simulink model "ssc_auto_ev_20b"  (R2020b)
settings: Solver=VariableStepAuto  StartTime=0.0  StopTime=200  RelTol=1e-3  AbsTol=1e-3
PreLoadFcn:
  | % Simulation parameters
  | dt = 0.01;
  | 
  | % Battery cell parameters
  | ssc_lithium_cell_1RC_ini
  | Nseries = 100;
  | Nparallel = 10;
  | 
  | % Motor parameters
  | max_torque = 220;
  | max_power = 80e3;
  | 
  | % Vehicle parameters
  | vehicle_mass = 4000;
  | wheel_radius = 0.35;
  | area = 5;
  | drag_coefficient = 0.25;
  | air_density = 1.225;
  | gravity = 9.81;
  | rolling_res_ratio = 0.015;
  | 
  | % Differential drive parameters
  | gear_ratio = 12;
  | 
  | % Simplified braking system parameters
  | force_max_pedal = 500;
  | braking_torque_to_pedal_force_ratio = -16;
  | 
  | % Vehicle controller parameters
  | hill_hold_max_speed = 0.5;
  | 
  | % Water properties for cooling circuit
  | load WaterProperties
  | 
  | % Input signals for Signal Editor block
  | load ssc_auto_ev_Inputs
values from neighbouring files (symbols this model uses):
  C1_LUT = [1913.6 4625.7 23306 10736 18036 12251 9022.9 12447 18872 40764 18721 33630 ... (21 elements, 7x3)]    [ssc_auto_ev_param.mat]
  Capacity_LUT = [28.0081 27.625 27.6392]    [ssc_auto_ev_param.mat]
  cell_Cp_heat = 810.5328    [ssc_auto_ev_param.mat]
  cell_mass = 1    [ssc_auto_ev_param.mat]
  Em_LUT = [3.4966 3.5519 3.6183 3.7066 3.9131 4.0748 4.1923 3.5057 3.566 3.6337 3.7127 3.9259 ... (21 elements, 7x3)]    [ssc_auto_ev_param.mat]
  Qe_init = 15.6845    [ssc_auto_ev_param.mat]
  R0_LUT = [0.0117 0.011 0.0114 0.0107 0.0107 0.0113 0.0116 0.0085 0.0085 0.0087 0.0082 0.0083 ... (21 elements, 7x3)]    [ssc_auto_ev_param.mat]
  R1_LUT = [0.0109 0.0069 0.0047 0.0034 0.0033 0.0033 0.0028 0.0029 0.0024 0.0026 0.0016 0.0023 ... (21 elements, 7x3)]    [ssc_auto_ev_param.mat]
  SOC_LUT = [0 0.1 0.25 0.5 0.75 0.9 1]    [ssc_auto_ev_param.mat]
  T_init = 293.15    [ssc_auto_ev_param.mat]
  Temperature_LUT = [278.15 293.15 313.15]    [ssc_auto_ev_param.mat]
undefined symbols (not defined in the file or in its folder): DiscIntNeverNeededParam, K, Lambda, tau, x0
libraries: fl_lib x656, nesl_utility x86, simulink x21, LiBatteryElements_lib x16, SignalEditorBlockLib x4, simulink_extras x4
(part 2 of 13)

== system ssc_auto_ev_20b/Step 2: Multirate Model ==
  note: The rotor iron thermal mass was pulled out of the
      | motor thermal model subsystem in Step 1 so that
      | it could be used to separate the thermal network
      | from the rest of the model in Step 2. Here, in Step 2,
      | it is replaced by a thermal mass network coupler
      | block from the Simscape Network Coupliers Library.
      | The same approach is used for the other motor and
      | the battery.
  note: There is no suitable existing model dynamic with
      | which to break the electrical connection to the battery.
      | Hence a network coupler block with internal voltage
      | and current sources is used which introduces its own
      | time constant. The electrical "+" connection of the
      | Motor Drive block has a series-connected current
      | source, and hence the voltage source in the coupler
      | block is connected to this port to avoid an invalid topology.
  note: The thermal circuit is set to run five times slower
      | than the control and vehicle dynamics subsystems.
      | It is often the case that the thermal time constants
      | are slower than the other domain time constants,
      | and so a longer sample time can be used.
  note: The battery subsystem is set to run two
      | times slower than the control and vehicle
      | dynamics subsystems. Battery time constants
      | are also typically slower than drive torque time
      | constants and mechanical time constants, and
      | so can be run with a larger sample time.
  note: Experimenting with the flexible
      | shaft coupler by using its Analysis
      | tab indicates that breaking the
      | network at this rotating shaft
      | is not a good idea. It would
      | require the sampling to be
      | increased to about 1000Hz to
      | track the design model.
  Battery : Subsystem  mask(Lithium cell (one RC-branch equivalent circuit)){Nseries=Nseries, Nparallel=Nparallel, Qe_init=Qe_init, T_init=T_init, Capacity_LUT=Capacity_LUT, Em_LUT=Em_LUT, R0_LUT=R0_LUT, R1_LUT=R1_LUT, C1_LUT=C1_LUT, cell_mass=cell_mass, cell_Cp_heat=cell_Cp_heat, SOC_LUT=SOC_LUT, Temperature_LUT=Temperature_LUT}
      mask prompts: Nseries "Number of series-connected parallel sets"; Nparallel "Number of parallel-connected cells per parallel set"; Qe_init "Initial cell charge deficit (A*hr)"; T_init "Initial cell temperature (K)"; Capacity_LUT "Capacity (A*hr, 1xN table)"; Em_LUT "Em open-circuit voltage, Em (volts, MxN table)"; R0_LUT "R0 terminal resistance (ohms, MxN table)"; R1_LUT "R1 cell resistance (ohms, MxN table)"; C1_LUT "C1 capacitance (farads, MxN table)"; cell_mass "Cell mass (kg)"; cell_Cp_heat "Cell specific heat (J/kg/K)"; SOC_LUT "SOC table breakpoints (Mx1 array)"; Temperature_LUT "Temperature table breakpoints (K, 1xN array)"
      mask DialogControl ParameterTabVar0 Prompt: Main
      mask DialogControl ParameterTabVar01 Prompt: Electrical (per cell)
      mask DialogControl ParameterTabVar012 Prompt: Thermal (per cell)
      mask DialogControl ParameterTabVar0123 Prompt: Table Breakpoints
      mask Display:
      | % Battery icon
      | plot([1.8 1.3],[0 0])
      | plot([-0.6 -1.6 -1.6 -2.2],[0 0 -0.9 -0.9])
      | patch([1 1 -1 -1]*0.15+0.7,[-1 1 1 -1]*0.4,[0;0;0]);
      | patch([1 1 -1 -1]*0.15-0.6,[-1 1 1 -1]*0.4,[0;0;0]);
      | patch([1 1 -1 -1]*0.15+1.3,[-1 1 1 -1]*0.8,[0;0;0]);
      | patch([1 1 -1 -1]*0.15-0.0,[-1 1 1 -1]*0.8,[0;0;0]);
      | % Thermal port
      | plot([-1.6,-1.3],[1.2,1.2])
      | plot([-1.6,-1.3],[0.5,0.5])
      | plot([-1.6,-2.5],[0.8,0.8])
      | plot(0.2*sin(0:2*pi/50:2*pi)-1.6,0.35*cos(0:2*pi/50:2*pi)+0.85)
      | plot(0.2*sin(0:2*pi/50:pi)-1.3,0.35*cos(0:2*pi/50:pi)+0.85)
      | 
      | % Plot points to set plot range
      | color('white');plot(2.5,1.5);plot(-2.5,-1.5)
  Battery Thermal Mass : Subsystem  mask(Network Coupler (Thermal Mass)){}
      mask init:
      | % Icon
      | %key = 'Simscape.NetworkCouplers.ThermalMass';
      | %foundation.internal.couplers.updateIcon(gcb,'thermalMass.svg',key)
      settings: OpenFcn=open_system(gcbh,'force')
      mask Help: web([docroot '/physmod/simscape/ref/networkcouplerthermalmass.html'])
      mask Display:
      | color('red');
      | port_label('LConn', 1,'1')
      | port_label('RConn', 1,'2')
  Cooling System : Subsystem  Tag=PublishSubsystem
      settings: PortSchema="{\"entries\":[{\"content\":{\"sides\":[{\"content\":{\"connectorIds\":[]},\"type\":\"ConnectorPlacement.EquallySpacedRectSide\",\"uuid\":\"d96bbf63-bcbb-4f3a-92bd-eaf78ab4538b\"},{\"content\":{\"connectorIds\":[],\"side\":\"RIGHT\"},\"type\":\"ConnectorPlacement.EquallySpacedRectSide\",\"uuid\":\"b082d3d3-6635-4bf9-9df2-69e4bab78a2b\"},{\"content\":{\"connectorIds\":[\"LConn1\"],\"side\":\"TOP\"},\"type\":\"ConnectorPlacement.EquallySpacedRectSide\",\"uuid\":\"f7177de9-9ba4-478b-b096-87cbc5cd4871\"},{\"content\":{\"connectorIds\":[\"RConn1\"],\"side\":\"BOTTOM\"},\"type\":\"ConnectorPlacement.EquallySpacedRectSide\",\"uuid\":\"4233a269-bfd6-4033-b1ed-0dae7bb50bca\"}]},\"type\":\"ConnectorPlacement.EquallySpacedConnector\",\"uuid\":\"6f10551f-62c9-4564-9ac9-7ef3b87c77d6\"}],\"packageUris\":[\"http://schema.mathworks.com/mf0/Connector/R2020b\"],\"version\":\"1.0\"}"
  Driver and Environment : Subsystem
  ERef1 : fl_lib/Electrical/Electrical Elements/Electrical Reference
      settings: SourceProductBaseCode=PW,SS,VE
  ERef2 : fl_lib/Electrical/Electrical Elements/Electrical Reference
      settings: SourceProductBaseCode=PW,SS,VE
  Environment : Subsystem
  Motor 1 Thermal Model : Subsystem
  Motor 2 Thermal Model : Subsystem
  Motor Drive : Subsystem  Tag=PublishSubsystem  VariantControl=Variant1
  Network Coupler (Flexible Shaft) : Subsystem  Commented=on  mask(Network Coupler (Flexible Shaft)){}
      mask init:
      | % Icon
      | key = 'Simscape.NetworkCouplers.FlexibleShaft';
      | foundation.internal.couplers.updateIcon(gcb,'flexibleShaft.svg',key)
      settings: OpenFcn=open_system(gcbh,'force')
      mask Help: web([docroot '/physmod/simscape/ref/networkcouplerflexibleshaft.html'])
      mask Display:
      | color('red');
      | port_label('LConn', 1,'1')
      | port_label('RConn', 1,'2')
  Network Coupler (Voltage-Current) : Subsystem  mask(Network Coupler (Voltage-Current)){}
      mask init:
      | % Icon
      | %key = 'Simscape.NetworkCouplers.ElectricalVoltageCurrent';
      | %foundation.internal.couplers.updateIcon(gcb,'voltageCurrentSource.svg',key)
      settings: OpenFcn=open_system(gcbh,'force')
      mask Help: web([docroot '/physmod/simscape/ref/networkcouplervoltagecurrent.html'])
      mask Display:
      | color('red');
      | port_label('LConn', 1,'1')
      | port_label('RConn', 1,'2')
  Rotor Iron Thermal Mass/1 : Subsystem  mask(Network Coupler (Thermal Mass)){}
      mask init:
      | % Icon
      | %key = 'Simscape.NetworkCouplers.ThermalMass';
      | %foundation.internal.couplers.updateIcon(gcb,'thermalMass.svg',key)
      settings: OpenFcn=open_system(gcbh,'force')
      mask Help: web([docroot '/physmod/simscape/ref/networkcouplerthermalmass.html'])
      mask Display:
      | color('red');
      | port_label('LConn', 1,'1')
      | port_label('RConn', 1,'2')
  Rotor Iron Thermal Mass/2 : Subsystem  mask(Network Coupler (Thermal Mass)){}
      mask init:
      | % Icon
      | %key = 'Simscape.NetworkCouplers.ThermalMass';
      | %foundation.internal.couplers.updateIcon(gcb,'thermalMass.svg',key)
      settings: OpenFcn=open_system(gcbh,'force')
      mask Help: web([docroot '/physmod/simscape/ref/networkcouplerthermalmass.html'])
      mask Display:
      | color('red');
      | port_label('LConn', 1,'1')
      | port_label('RConn', 1,'2')
  Solver Configuration1 : nesl_utility/Solver Configuration  PhysicalDomain=network_engine_domain  SubClassName=solver  LeftPortType=input  RightPortType=generic  Tones=[]  Harmonics=[]  SimulateNoise=off  Profile=off  UseLocalSampling=off  EnableSwitchedLinearOptims=on  FrequencyDomain=off  UseCCode=off  RelTol=0.001  AbsTol=1e-06  MinStep=1e-09  ToWorkspace=off  RevertToSquareIcSolve=off  NumHomotopyIterations=100  PhasorMode=off  PhasorModeNumHarmonics=1  DoDC=off  ResidualTolerance=1e-9  UseLocalSolver=on  LocalSolverChoice=NE_BACKWARD_EULER_ADVANCER  LocalSolverSampleTime=dt  DoFixedCost=on  MaxNonlinIter=3  MaxModeIter=2  ComputeImpulses=off  ImpulseIterations=2  LinearAlgebra=auto  EquationFormulation=NE_TIME_EF  DelaysMemoryBudget=1024  AutomaticFiltering=on  FilteringTimeConstant=0.001  PartitionStorageMethod=AS_NEEDED  PartitionMemoryBudget=1024  PartitionMethod=FAST
      settings: AttributesFormatString=Local Solver: %<UseLocalSolver>  SourceProductBaseCode=SS,PW,VE
  Solver Configuration2 : nesl_utility/Solver Configuration  PhysicalDomain=network_engine_domain  SubClassName=solver  LeftPortType=input  RightPortType=generic  Tones=[]  Harmonics=[]  SimulateNoise=off  Profile=off  UseLocalSampling=off  EnableSwitchedLinearOptims=on  FrequencyDomain=off  UseCCode=off  RelTol=0.001  AbsTol=1e-06  MinStep=1e-09  ToWorkspace=off  RevertToSquareIcSolve=off  NumHomotopyIterations=100  PhasorMode=off  PhasorModeNumHarmonics=1  DoDC=off  ResidualTolerance=1e-9  UseLocalSolver=on  LocalSolverChoice=NE_BACKWARD_EULER_ADVANCER  LocalSolverSampleTime=dt*5  DoFixedCost=on  MaxNonlinIter=3  MaxModeIter=2  ComputeImpulses=off  ImpulseIterations=2  LinearAlgebra=auto  EquationFormulation=NE_TIME_EF  DelaysMemoryBudget=1024  AutomaticFiltering=on  FilteringTimeConstant=0.001  PartitionStorageMethod=AS_NEEDED  PartitionMemoryBudget=1024  PartitionMethod=FAST
      settings: AttributesFormatString=Local Solver: %<UseLocalSolver>  SourceProductBaseCode=SS,PW,VE
  Solver Configuration3 : nesl_utility/Solver Configuration  PhysicalDomain=network_engine_domain  SubClassName=solver  LeftPortType=input  RightPortType=generic  Tones=[]  Harmonics=[]  SimulateNoise=off  Profile=off  UseLocalSampling=off  EnableSwitchedLinearOptims=on  FrequencyDomain=off  UseCCode=off  RelTol=0.001  AbsTol=1e-06  MinStep=1e-09  ToWorkspace=off  RevertToSquareIcSolve=off  NumHomotopyIterations=100  PhasorMode=off  PhasorModeNumHarmonics=1  DoDC=off  ResidualTolerance=1e-9  UseLocalSolver=on  LocalSolverChoice=NE_BACKWARD_EULER_ADVANCER  LocalSolverSampleTime=dt*2  DoFixedCost=on  MaxNonlinIter=3  MaxModeIter=2  ComputeImpulses=off  ImpulseIterations=2  LinearAlgebra=auto  EquationFormulation=NE_TIME_EF  DelaysMemoryBudget=1024  AutomaticFiltering=on  FilteringTimeConstant=0.001  PartitionStorageMethod=AS_NEEDED  PartitionMemoryBudget=1024  PartitionMethod=FAST
      settings: AttributesFormatString=Local Solver: %<UseLocalSolver>  SourceProductBaseCode=SS,PW,VE
  Unit Delay1 : UnitDelay  SampleTime=dt  HasFrameUpgradeWarning=on
  Vehicle Dynamics : Subsystem
  Vehicle Control : Subsystem  Tag=PublishSubsystem
      settings: PortSchema="{\"entries\":[{\"content\":{\"sides\":[{\"content\":{\"connectorIds\":[\"In1\"]},\"type\":\"ConnectorPlacement.EquallySpacedRectSide\",\"uuid\":\"b68a5c30-2a17-4a0c-a85e-064518f12190\"},{\"content\":{\"connectorIds\":[\"In2\",\"Out1\"],\"side\":\"RIGHT\"},\"type\":\"ConnectorPlacement.EquallySpacedRectSide\",\"uuid\":\"e14e894a-37e1-47c1-8ef8-e46ccf22e5bb\"},{\"content\":{\"connectorIds\":[],\"side\":\"TOP\"},\"type\":\"ConnectorPlacement.EquallySpacedRectSide\",\"uuid\":\"6e722464-54b7-4a5f-a776-dae3a11285e7\"}]},\"type\":\"ConnectorPlacement.EquallySpacedConnector\",\"uuid\":\"82601a10-23cc-4178-a2d7-02b0e1b6e975\"}],\"packageUris\":[\"http://schema.mathworks.com/mf0/Connector/R2020b\"],\"version\":\"1.0\"}"
  ZOH/1 : ZeroOrderHold  SampleTime=dt
  wires:
  Driver and Environment/2(ECU) -> Vehicle Control/1(ECU)
  ZOH/1/1 -> Vehicle Control/2(wMeas)
  Vehicle Control/1(iRef) -> Unit Delay1/1
  Motor Drive/1(w) -> ZOH/1/1
  Driver and Environment/1(Veh) -> Vehicle Dynamics/1(Test data)
  Driver and Environment/3(Env) -> Environment/1(T)
  Unit Delay1/1 -> Motor Drive/1(iRef)
  connections:
  ERef1/LConn1 -- Solver Configuration3/RConn1 -- Battery/LConn2
  Solver Configuration1/RConn1 -- Motor Drive/RConn1 -- Vehicle Dynamics/LConn1
  Cooling System/RConn1 -- Motor 1 Thermal Model/LConn1 -- Motor 2 Thermal Model/LConn1 -- Solver Configuration2/RConn1 -- Environment/RConn1
  ERef2/LConn1 -- Motor Drive/LConn2
  Cooling System/LConn1 -- Battery Thermal Mass/RConn1
  Battery Thermal Mass/LConn1 -- Battery/LConn1
  Network Coupler (Voltage-Current)/RConn1 -- Battery/RConn1
  Network Coupler (Voltage-Current)/LConn1 -- Motor Drive/LConn1
  Motor 2 Thermal Model/RConn1 -- Rotor Iron Thermal Mass/2/RConn1
  Rotor Iron Thermal Mass/2/LConn1 -- Motor Drive/LConn4
  Motor 1 Thermal Model/RConn1 -- Rotor Iron Thermal Mass/1/RConn1
  Rotor Iron Thermal Mass/1/LConn1 -- Motor Drive/LConn3

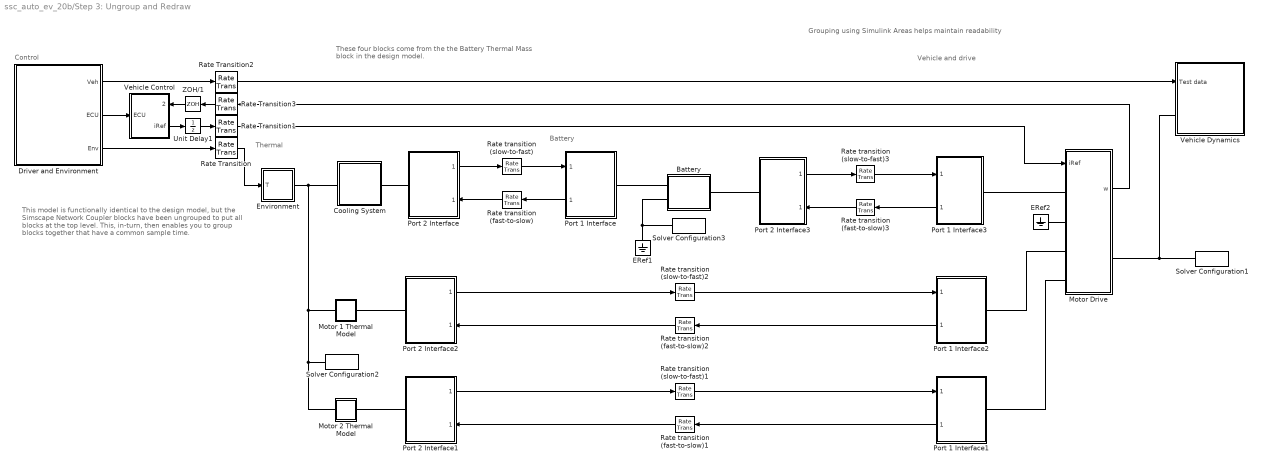
== system ssc_auto_ev_20b/Step 3: Ungroup and Redraw ==
  note: This model is functionally identical to the design model, but
      | the Simscape Network Coupler blocks have been ungrouped
      | to put all blocks at the top level. This, in-turn, then enables
      | you to group blocks together that have a common sample time.
  note: Thermal
  note: Battery
  note: Vehicle and drive
  note: Control
  note: These four blocks come from the the Battery Thermal Mass
      | block in the design model.
  note: Grouping using Simulink Areas helps maintain readability
  Battery : Subsystem  mask(Lithium cell (one RC-branch equivalent circuit)){Nseries=Nseries, Nparallel=Nparallel, Qe_init=Qe_init, T_init=T_init, Capacity_LUT=Capacity_LUT, Em_LUT=Em_LUT, R0_LUT=R0_LUT, R1_LUT=R1_LUT, C1_LUT=C1_LUT, cell_mass=cell_mass, cell_Cp_heat=cell_Cp_heat, SOC_LUT=SOC_LUT, Temperature_LUT=Temperature_LUT}
      mask prompts: Nseries "Number of series-connected parallel sets"; Nparallel "Number of parallel-connected cells per parallel set"; Qe_init "Initial cell charge deficit (A*hr)"; T_init "Initial cell temperature (K)"; Capacity_LUT "Capacity (A*hr, 1xN table)"; Em_LUT "Em open-circuit voltage, Em (volts, MxN table)"; R0_LUT "R0 terminal resistance (ohms, MxN table)"; R1_LUT "R1 cell resistance (ohms, MxN table)"; C1_LUT "C1 capacitance (farads, MxN table)"; cell_mass "Cell mass (kg)"; cell_Cp_heat "Cell specific heat (J/kg/K)"; SOC_LUT "SOC table breakpoints (Mx1 array)"; Temperature_LUT "Temperature table breakpoints (K, 1xN array)"
      mask DialogControl ParameterTabVar0 Prompt: Main
      mask DialogControl ParameterTabVar01 Prompt: Electrical (per cell)
      mask DialogControl ParameterTabVar012 Prompt: Thermal (per cell)
      mask DialogControl ParameterTabVar0123 Prompt: Table Breakpoints
      mask Display:
      | % Battery icon
      | plot([1.8 1.3],[0 0])
      | plot([-0.6 -1.6 -1.6 -2.2],[0 0 -0.9 -0.9])
      | patch([1 1 -1 -1]*0.15+0.7,[-1 1 1 -1]*0.4,[0;0;0]);
      | patch([1 1 -1 -1]*0.15-0.6,[-1 1 1 -1]*0.4,[0;0;0]);
      | patch([1 1 -1 -1]*0.15+1.3,[-1 1 1 -1]*0.8,[0;0;0]);
      | patch([1 1 -1 -1]*0.15-0.0,[-1 1 1 -1]*0.8,[0;0;0]);
      | % Thermal port
      | plot([-1.6,-1.3],[1.2,1.2])
      | plot([-1.6,-1.3],[0.5,0.5])
      | plot([-1.6,-2.5],[0.8,0.8])
      | plot(0.2*sin(0:2*pi/50:2*pi)-1.6,0.35*cos(0:2*pi/50:2*pi)+0.85)
      | plot(0.2*sin(0:2*pi/50:pi)-1.3,0.35*cos(0:2*pi/50:pi)+0.85)
      | 
      | % Plot points to set plot range
      | color('white');plot(2.5,1.5);plot(-2.5,-1.5)
  Cooling System : Subsystem  Tag=PublishSubsystem
      settings: PortSchema="{\"entries\":[{\"content\":{\"sides\":[{\"content\":{\"connectorIds\":[]},\"type\":\"ConnectorPlacement.EquallySpacedRectSide\",\"uuid\":\"d96bbf63-bcbb-4f3a-92bd-eaf78ab4538b\"},{\"content\":{\"connectorIds\":[],\"side\":\"RIGHT\"},\"type\":\"ConnectorPlacement.EquallySpacedRectSide\",\"uuid\":\"b082d3d3-6635-4bf9-9df2-69e4bab78a2b\"},{\"content\":{\"connectorIds\":[\"LConn1\"],\"side\":\"TOP\"},\"type\":\"ConnectorPlacement.EquallySpacedRectSide\",\"uuid\":\"f7177de9-9ba4-478b-b096-87cbc5cd4871\"},{\"content\":{\"connectorIds\":[\"RConn1\"],\"side\":\"BOTTOM\"},\"type\":\"ConnectorPlacement.EquallySpacedRectSide\",\"uuid\":\"4233a269-bfd6-4033-b1ed-0dae7bb50bca\"}]},\"type\":\"ConnectorPlacement.EquallySpacedConnector\",\"uuid\":\"6f10551f-62c9-4564-9ac9-7ef3b87c77d6\"}],\"packageUris\":[\"http://schema.mathworks.com/mf0/Connector/R2020b\"],\"version\":\"1.0\"}"
  Driver and Environment : Subsystem
  ERef1 : fl_lib/Electrical/Electrical Elements/Electrical Reference
      settings: SourceProductBaseCode=PW,SS,VE
  ERef2 : fl_lib/Electrical/Electrical Elements/Electrical Reference
      settings: SourceProductBaseCode=PW,SS,VE
  Environment : Subsystem
  Motor 1 Thermal Model : Subsystem
  Motor 2 Thermal Model : Subsystem
  Motor Drive : Subsystem  Tag=PublishSubsystem  VariantControl=Variant1
  Port 1 Interface : Subsystem  mask(Network Coupler (Thermal Mass) Port 1 Interface){thermalMass=cell_mass*Nseries*Nparallel*cell_Cp_heat, samplingType=physmod:simscape:couplers:SimscapeNetworkCouplersLib:VariableStepAtPorts1And2_PV, h1=dt*2, h2=dt*5, predictionDiscreteToContinuous=off, smoothingContinuousToDiscrete=off, predictionSlowToFast=off, smoothingFastToSlow=off, nSmooth=1, tsSmoothing=0.01, thermalConductanceNetwork=1, hRecommended=0.001, T0=T_init}
      mask prompts: thermalMass "physmod:simscape:couplers:SimscapeNetworkCouplersLib:ThermalMassJK_MP"; samplingType "physmod:simscape:couplers:SimscapeNetworkCouplersLib:SamplingType_MP"; h1 "physmod:simscape:couplers:SimscapeNetworkCouplersLib:Port1NetworkDiscreteSampleTimes_MP"; h2 "physmod:simscape:couplers:SimscapeNetworkCouplersLib:Port2NetworkDiscreteSampleTimes_MP"; predictionDiscreteToContinuous "physmod:simscape:couplers:SimscapeNetworkCouplersLib:UsePredictionWhenConnectingFixedStepToVariableStep_MP"; smoothingContinuousToDiscrete "physmod:simscape:couplers:SimscapeNetworkCouplersLib:UseSmoothingWhenConnectingVariableStepToFixedStep_MP"; predictionSlowToFast "physmod:simscape:couplers:SimscapeNetworkCouplersLib:UsePredictionWhenConnectingSlowToFastSampleTimes_MP"; smoothingFastToSlow "physmod:simscape:couplers:SimscapeNetworkCouplersLib:UseSmoothingWhenConnectingFastToSlowSampleTimes_MP"; nSmooth "physmod:simscape:couplers:SimscapeNetworkCouplersLib:NumberOfSamplesOverWhichToSmooth_MP"; tsSmoothing "physmod:simscape:couplers:SimscapeNetworkCouplersLib:SmoothingTimeConstants_MP"; thermalConductanceNetwork "physmod:simscape:couplers:SimscapeNetworkCouplersLib:ApproximateConnectedNetworkThermalConductanceWK_MP"; hRecommended "physmod:simscape:couplers:SimscapeNetworkCouplersLib:RecommendedMaxDiscreteSampleTimes_MP"; T0 "physmod:simscape:couplers:SimscapeNetworkCouplersLib:InitialTemperatureK_MP"
      mask help: physmod:simscape:couplers:SimscapeNetworkCouplersLib:NetworkCouplerThermalMassPort1Interface_MD
      mask init:
      | % Fixed step sample time value check
      | foundation.internal.couplers.checkSampleTimes(gcb,h1,h2);
      | 
      | % Remaining parameter value checks
      | foundation.internal.couplers.thermal.checkParametersThermalMass(thermalMass,T0);
      settings: PortSchema="{\"entries\":[{\"content\":{\"sides\":[{\"content\":{\"connectorIds\":[\"LConn1\"]},\"type\":\"ConnectorPlacement.EquallySpacedRectSide\",\"uuid\":\"a6d4a9fd-b5aa-40dc-ab7e-2b646b9b57bc\"},{\"content\":{\"connectorIds\":[\"Out1\",\"In1\"],\"side\":\"RIGHT\"},\"type\":\"ConnectorPlacement.EquallySpacedRectSide\",\"uuid\":\"31bb6273-5b9b-48d0-a1a2-6fbacb979b97\"},{\"content\":{\"connectorIds\":[],\"side\":\"TOP\"},\"type\":\"ConnectorPlacement.EquallySpacedRectSide\",\"uuid\":\"0f7afab2-4481-486c-9ad0-2b42c5b091a4\"}]},\"type\":\"ConnectorPlacement.EquallySpacedConnector\",\"uuid\":\"a98e47aa-cbfd-441a-b14c-c9ea515c056e\"}],\"packageUris\":[\"http://schema.mathworks.com/mf0/Connector/R2020b\"],\"version\":\"1.0\"}"
      mask Help: web([docroot '/physmod/simscape/ref/networkcouplerthermalmass.html'])
      mask TypeOptions samplingType: physmod:simscape:couplers:SimscapeNetworkCouplersLib:VariableStepAtPorts1And2_PV | physmod:simscape:couplers:SimscapeNetworkCouplersLib:VariableStepAtPort1AndFixedStepAtPort2_PV | physmod:simscape:couplers:SimscapeNetworkCouplersLib:FixedStepBothPortsWithCommonSampleTime_PV | physmod:simscape:couplers:SimscapeNetworkCouplersLib:FixedStepBothPortsWithFasterSamplingAtPort1_PV
      mask Callback samplingType: foundation.internal.couplers.thermal.parameterVisibilitiesThermalMass(gcb)
      mask Callback predictionDiscreteToContinuous: foundation.internal.couplers.thermal.parameterVisibilitiesThermalMass(gcb)
      mask Callback smoothingContinuousToDiscrete: foundation.internal.couplers.thermal.parameterVisibilitiesThermalMass(gcb)
      mask Callback predictionSlowToFast: foundation.internal.couplers.thermal.parameterVisibilitiesThermalMass(gcb)
      mask Callback smoothingFastToSlow: foundation.internal.couplers.thermal.parameterVisibilitiesThermalMass(gcb)
      mask DialogControl Main Prompt: Main
      mask DialogControl Analysis Prompt: Analysis
      mask DialogControl connectedNetworkInfo Prompt: Connected network information
      mask DialogControl derivedValues Prompt: Derived values
      mask DialogControl updateRecommendations Prompt: Update
      mask DialogControl updateRecommendations Callback: foundation.internal.couplers.thermal.analysisThermalMass(gcb);
      mask DialogControl InitialConditions Prompt: Initial Conditions
  Port 1 Interface1 : Subsystem  mask(Network Coupler (Thermal Mass) Port 1 Interface){thermalMass=10*447, samplingType=physmod:simscape:couplers:SimscapeNetworkCouplersLib:VariableStepAtPorts1And2_PV, h1=dt, h2=dt*5, predictionDiscreteToContinuous=off, smoothingContinuousToDiscrete=off, predictionSlowToFast=off, smoothingFastToSlow=off, nSmooth=1, tsSmoothing=0.01, thermalConductanceNetwork=1, hRecommended=0.001, T0=T_init}
      mask prompts: thermalMass "physmod:simscape:couplers:SimscapeNetworkCouplersLib:ThermalMassJK_MP"; samplingType "physmod:simscape:couplers:SimscapeNetworkCouplersLib:SamplingType_MP"; h1 "physmod:simscape:couplers:SimscapeNetworkCouplersLib:Port1NetworkDiscreteSampleTimes_MP"; h2 "physmod:simscape:couplers:SimscapeNetworkCouplersLib:Port2NetworkDiscreteSampleTimes_MP"; predictionDiscreteToContinuous "physmod:simscape:couplers:SimscapeNetworkCouplersLib:UsePredictionWhenConnectingFixedStepToVariableStep_MP"; smoothingContinuousToDiscrete "physmod:simscape:couplers:SimscapeNetworkCouplersLib:UseSmoothingWhenConnectingVariableStepToFixedStep_MP"; predictionSlowToFast "physmod:simscape:couplers:SimscapeNetworkCouplersLib:UsePredictionWhenConnectingSlowToFastSampleTimes_MP"; smoothingFastToSlow "physmod:simscape:couplers:SimscapeNetworkCouplersLib:UseSmoothingWhenConnectingFastToSlowSampleTimes_MP"; nSmooth "physmod:simscape:couplers:SimscapeNetworkCouplersLib:NumberOfSamplesOverWhichToSmooth_MP"; tsSmoothing "physmod:simscape:couplers:SimscapeNetworkCouplersLib:SmoothingTimeConstants_MP"; thermalConductanceNetwork "physmod:simscape:couplers:SimscapeNetworkCouplersLib:ApproximateConnectedNetworkThermalConductanceWK_MP"; hRecommended "physmod:simscape:couplers:SimscapeNetworkCouplersLib:RecommendedMaxDiscreteSampleTimes_MP"; T0 "physmod:simscape:couplers:SimscapeNetworkCouplersLib:InitialTemperatureK_MP"
      mask help: physmod:simscape:couplers:SimscapeNetworkCouplersLib:NetworkCouplerThermalMassPort1Interface_MD
      mask init:
      | % Fixed step sample time value check
      | %foundation.internal.couplers.checkSampleTimes(gcb,h1,h2);
      | 
      | % Remaining parameter value checks
      | %foundation.internal.couplers.thermal.checkParametersThermalMass(thermalMass,T0);
      settings: PortSchema="{\"entries\":[{\"content\":{\"sides\":[{\"content\":{\"connectorIds\":[\"LConn1\"]},\"type\":\"ConnectorPlacement.EquallySpacedRectSide\",\"uuid\":\"a6d4a9fd-b5aa-40dc-ab7e-2b646b9b57bc\"},{\"content\":{\"connectorIds\":[\"Out1\",\"In1\"],\"side\":\"RIGHT\"},\"type\":\"ConnectorPlacement.EquallySpacedRectSide\",\"uuid\":\"31bb6273-5b9b-48d0-a1a2-6fbacb979b97\"},{\"content\":{\"connectorIds\":[],\"side\":\"TOP\"},\"type\":\"ConnectorPlacement.EquallySpacedRectSide\",\"uuid\":\"0f7afab2-4481-486c-9ad0-2b42c5b091a4\"}]},\"type\":\"ConnectorPlacement.EquallySpacedConnector\",\"uuid\":\"a98e47aa-cbfd-441a-b14c-c9ea515c056e\"}],\"packageUris\":[\"http://schema.mathworks.com/mf0/Connector/R2020b\"],\"version\":\"1.0\"}"
      mask Help: web([docroot '/physmod/simscape/ref/networkcouplerthermalmass.html'])
      mask TypeOptions samplingType: physmod:simscape:couplers:SimscapeNetworkCouplersLib:VariableStepAtPorts1And2_PV | physmod:simscape:couplers:SimscapeNetworkCouplersLib:VariableStepAtPort1AndFixedStepAtPort2_PV | physmod:simscape:couplers:SimscapeNetworkCouplersLib:FixedStepBothPortsWithCommonSampleTime_PV | physmod:simscape:couplers:SimscapeNetworkCouplersLib:FixedStepBothPortsWithFasterSamplingAtPort1_PV
      mask Callback samplingType: foundation.internal.couplers.thermal.parameterVisibilitiesThermalMass(gcb)
      mask Callback predictionDiscreteToContinuous: foundation.internal.couplers.thermal.parameterVisibilitiesThermalMass(gcb)
      mask Callback smoothingContinuousToDiscrete: foundation.internal.couplers.thermal.parameterVisibilitiesThermalMass(gcb)
      mask Callback predictionSlowToFast: foundation.internal.couplers.thermal.parameterVisibilitiesThermalMass(gcb)
      mask Callback smoothingFastToSlow: foundation.internal.couplers.thermal.parameterVisibilitiesThermalMass(gcb)
      mask DialogControl Main Prompt: Main
      mask DialogControl Analysis Prompt: Analysis
      mask DialogControl connectedNetworkInfo Prompt: Connected network information
      mask DialogControl derivedValues Prompt: Derived values
      mask DialogControl updateRecommendations Prompt: Update
      mask DialogControl updateRecommendations Callback: foundation.internal.couplers.thermal.analysisThermalMass(gcb);
      mask DialogControl InitialConditions Prompt: Initial Conditions
  Port 1 Interface2 : Subsystem  mask(Network Coupler (Thermal Mass) Port 1 Interface){thermalMass=10*447, samplingType=physmod:simscape:couplers:SimscapeNetworkCouplersLib:VariableStepAtPorts1And2_PV, h1=dt, h2=dt*5, predictionDiscreteToContinuous=off, smoothingContinuousToDiscrete=off, predictionSlowToFast=off, smoothingFastToSlow=off, nSmooth=1, tsSmoothing=0.01, thermalConductanceNetwork=1, hRecommended=0.001, T0=T_init}
      mask prompts: thermalMass "physmod:simscape:couplers:SimscapeNetworkCouplersLib:ThermalMassJK_MP"; samplingType "physmod:simscape:couplers:SimscapeNetworkCouplersLib:SamplingType_MP"; h1 "physmod:simscape:couplers:SimscapeNetworkCouplersLib:Port1NetworkDiscreteSampleTimes_MP"; h2 "physmod:simscape:couplers:SimscapeNetworkCouplersLib:Port2NetworkDiscreteSampleTimes_MP"; predictionDiscreteToContinuous "physmod:simscape:couplers:SimscapeNetworkCouplersLib:UsePredictionWhenConnectingFixedStepToVariableStep_MP"; smoothingContinuousToDiscrete "physmod:simscape:couplers:SimscapeNetworkCouplersLib:UseSmoothingWhenConnectingVariableStepToFixedStep_MP"; predictionSlowToFast "physmod:simscape:couplers:SimscapeNetworkCouplersLib:UsePredictionWhenConnectingSlowToFastSampleTimes_MP"; smoothingFastToSlow "physmod:simscape:couplers:SimscapeNetworkCouplersLib:UseSmoothingWhenConnectingFastToSlowSampleTimes_MP"; nSmooth "physmod:simscape:couplers:SimscapeNetworkCouplersLib:NumberOfSamplesOverWhichToSmooth_MP"; tsSmoothing "physmod:simscape:couplers:SimscapeNetworkCouplersLib:SmoothingTimeConstants_MP"; thermalConductanceNetwork "physmod:simscape:couplers:SimscapeNetworkCouplersLib:ApproximateConnectedNetworkThermalConductanceWK_MP"; hRecommended "physmod:simscape:couplers:SimscapeNetworkCouplersLib:RecommendedMaxDiscreteSampleTimes_MP"; T0 "physmod:simscape:couplers:SimscapeNetworkCouplersLib:InitialTemperatureK_MP"
      mask help: physmod:simscape:couplers:SimscapeNetworkCouplersLib:NetworkCouplerThermalMassPort1Interface_MD
      mask init: same as ssc_auto_ev_20b/Step 3: Ungroup and Redraw/Port 1 Interface1
      settings: PortSchema="{\"entries\":[{\"content\":{\"sides\":[{\"content\":{\"connectorIds\":[\"LConn1\"]},\"type\":\"ConnectorPlacement.EquallySpacedRectSide\",\"uuid\":\"a6d4a9fd-b5aa-40dc-ab7e-2b646b9b57bc\"},{\"content\":{\"connectorIds\":[\"Out1\",\"In1\"],\"side\":\"RIGHT\"},\"type\":\"ConnectorPlacement.EquallySpacedRectSide\",\"uuid\":\"31bb6273-5b9b-48d0-a1a2-6fbacb979b97\"},{\"content\":{\"connectorIds\":[],\"side\":\"TOP\"},\"type\":\"ConnectorPlacement.EquallySpacedRectSide\",\"uuid\":\"0f7afab2-4481-486c-9ad0-2b42c5b091a4\"}]},\"type\":\"ConnectorPlacement.EquallySpacedConnector\",\"uuid\":\"a98e47aa-cbfd-441a-b14c-c9ea515c056e\"}],\"packageUris\":[\"http://schema.mathworks.com/mf0/Connector/R2020b\"],\"version\":\"1.0\"}"
      mask Help: web([docroot '/physmod/simscape/ref/networkcouplerthermalmass.html'])
      mask TypeOptions samplingType: physmod:simscape:couplers:SimscapeNetworkCouplersLib:VariableStepAtPorts1And2_PV | physmod:simscape:couplers:SimscapeNetworkCouplersLib:VariableStepAtPort1AndFixedStepAtPort2_PV | physmod:simscape:couplers:SimscapeNetworkCouplersLib:FixedStepBothPortsWithCommonSampleTime_PV | physmod:simscape:couplers:SimscapeNetworkCouplersLib:FixedStepBothPortsWithFasterSamplingAtPort1_PV
      mask Callback samplingType: foundation.internal.couplers.thermal.parameterVisibilitiesThermalMass(gcb)
      mask Callback predictionDiscreteToContinuous: foundation.internal.couplers.thermal.parameterVisibilitiesThermalMass(gcb)
      mask Callback smoothingContinuousToDiscrete: foundation.internal.couplers.thermal.parameterVisibilitiesThermalMass(gcb)
      mask Callback predictionSlowToFast: foundation.internal.couplers.thermal.parameterVisibilitiesThermalMass(gcb)
      mask Callback smoothingFastToSlow: foundation.internal.couplers.thermal.parameterVisibilitiesThermalMass(gcb)
      mask DialogControl Main Prompt: Main
      mask DialogControl Analysis Prompt: Analysis
      mask DialogControl connectedNetworkInfo Prompt: Connected network information
      mask DialogControl derivedValues Prompt: Derived values
      mask DialogControl updateRecommendations Prompt: Update
      mask DialogControl updateRecommendations Callback: foundation.internal.couplers.thermal.analysisThermalMass(gcb);
      mask DialogControl InitialConditions Prompt: Initial Conditions
  Port 1 Interface3 : Subsystem  mask(Network Coupler (Voltage-Current) Port 1 Interface){samplingType=physmod:simscape:couplers:SimscapeNetworkCouplersLib:VariableStepAtPorts1And2_PV, ts=1e-3, h1=dt, h2=dt*2, predictionDiscreteToContinuous=off, smoothingContinuousToDiscrete=off, predictionSlowToFast=off, smoothingFastToSlow=off, nSmooth=1, tsSmoothing=0.01, tsMax=1, tau=0.2, i0=0, v0=0}
      mask prompts: samplingType "physmod:simscape:couplers:SimscapeNetworkCouplersLib:SamplingType_MP"; ts "physmod:simscape:couplers:SimscapeNetworkCouplersLib:SeparatorTimeConstants_MP"; h1 "physmod:simscape:couplers:SimscapeNetworkCouplersLib:Port1NetworkDiscreteSampleTimes_MP"; h2 "physmod:simscape:couplers:SimscapeNetworkCouplersLib:Port2NetworkDiscreteSampleTimes_MP"; predictionDiscreteToContinuous "physmod:simscape:couplers:SimscapeNetworkCouplersLib:UsePredictionWhenConnectingFixedStepToVariableStep_MP"; smoothingContinuousToDiscrete "physmod:simscape:couplers:SimscapeNetworkCouplersLib:UseSmoothingWhenConnectingVariableStepToFixedStep_MP"; predictionSlowToFast "physmod:simscape:couplers:SimscapeNetworkCouplersLib:UsePredictionWhenConnectingSlowToFastSampleTimes_MP"; smoothingFastToSlow "physmod:simscape:couplers:SimscapeNetworkCouplersLib:UseSmoothingWhenConnectingFastToSlowSampleTimes_MP"; nSmooth "physmod:simscape:couplers:SimscapeNetworkCouplersLib:NumberOfSamplesOverWhichToSmooth_MP"; tsSmoothing "physmod:simscape:couplers:SimscapeNetworkCouplersLib:SmoothingTimeConstants_MP"; tsMax "physmod:simscape:couplers:SimscapeNetworkCouplersLib:CalculatedFastestTrackableTimeConstants_MP"; tau "physmod:simscape:couplers:SimscapeNetworkCouplersLib:CalculatedFilterTimeConstants_MP"; i0 "physmod:simscape:couplers:SimscapeNetworkCouplersLib:InitialCurrentA_MP"; v0 "physmod:simscape:couplers:SimscapeNetworkCouplersLib:InitialVoltageV_MP"
      mask help:
      | Port 1 interface for use when breaking two Simscape(TM) networks at an electrical connection. A first-order filter is used to break algebraic constraints between the two networks.
      |
      | Connect Port 1 to the network with the higher sample rate, or the network that is variable step if interfacing fixed step and variable step networks.
      mask init:
      | % Fixed step sample time value check
      | foundation.internal.couplers.checkSampleTimes(gcb,h1,h2);
      | 
      | % Derived parameters
      | [tau,tsMax] = foundation.internal.couplers.electrical.derivedParamsSources(gcb,ts,h1,h2);
      settings: PortSchema="{\"entries\":[{\"content\":{\"sides\":[{\"content\":{\"connectorIds\":[\"LConn1\"]},\"type\":\"ConnectorPlacement.EquallySpacedRectSide\",\"uuid\":\"a6d4a9fd-b5aa-40dc-ab7e-2b646b9b57bc\"},{\"content\":{\"connectorIds\":[\"Out1\",\"In1\"],\"side\":\"RIGHT\"},\"type\":\"ConnectorPlacement.EquallySpacedRectSide\",\"uuid\":\"31bb6273-5b9b-48d0-a1a2-6fbacb979b97\"},{\"content\":{\"connectorIds\":[],\"side\":\"TOP\"},\"type\":\"ConnectorPlacement.EquallySpacedRectSide\",\"uuid\":\"0f7afab2-4481-486c-9ad0-2b42c5b091a4\"}]},\"type\":\"ConnectorPlacement.EquallySpacedConnector\",\"uuid\":\"a98e47aa-cbfd-441a-b14c-c9ea515c056e\"}],\"packageUris\":[\"http://schema.mathworks.com/mf0/Connector/R2020b\"],\"version\":\"1.0\"}"
      mask Help: web([docroot '/physmod/simscape/ref/networkcouplervoltagecurrent.html'])
      mask TypeOptions samplingType: physmod:simscape:couplers:SimscapeNetworkCouplersLib:VariableStepAtPorts1And2_PV | physmod:simscape:couplers:SimscapeNetworkCouplersLib:VariableStepAtPort1AndFixedStepAtPort2_PV | physmod:simscape:couplers:SimscapeNetworkCouplersLib:FixedStepBothPortsWithCommonSampleTime_PV | physmod:simscape:couplers:SimscapeNetworkCouplersLib:FixedStepBothPortsWithFasterSamplingAtPort1_PV
      mask Callback samplingType: foundation.internal.couplers.electrical.parameterVisibilitiesSources(gcb)
      mask Callback predictionDiscreteToContinuous: foundation.internal.couplers.electrical.parameterVisibilitiesSources(gcb)
      mask Callback smoothingContinuousToDiscrete: foundation.internal.couplers.electrical.parameterVisibilitiesSources(gcb)
      mask Callback predictionSlowToFast: foundation.internal.couplers.electrical.parameterVisibilitiesSources(gcb)
      mask Callback smoothingFastToSlow: foundation.internal.couplers.electrical.parameterVisibilitiesSources(gcb)
      mask DialogControl Main Prompt: Main
      mask DialogControl Analysis Prompt: Analysis
      mask DialogControl updateRecommendations Prompt: Update
      mask DialogControl updateRecommendations Callback: foundation.internal.couplers.electrical.analysisSources(gcb);
      mask DialogControl InitialConditions Prompt: Initial Conditions
  Port 2 Interface : Subsystem  mask(Network Coupler (Thermal Mass) Port 2 Interface){}
      mask help: physmod:simscape:couplers:SimscapeNetworkCouplersLib:NetworkCouplerThermalMassPort2Interface_MD
      settings: PortSchema="{\"entries\":[{\"content\":{\"sides\":[{\"content\":{\"connectorIds\":[\"In1\",\"Out1\"]},\"type\":\"ConnectorPlacement.EquallySpacedRectSide\",\"uuid\":\"5a4c1550-e77d-42df-bf3e-b81963920de7\"},{\"content\":{\"connectorIds\":[\"RConn1\"],\"side\":\"RIGHT\"},\"type\":\"ConnectorPlacement.EquallySpacedRectSide\",\"uuid\":\"3fd730f7-5937-4563-a365-595aaae9027b\"},{\"content\":{\"connectorIds\":[],\"side\":\"TOP\"},\"type\":\"ConnectorPlacement.EquallySpacedRectSide\",\"uuid\":\"c16e04e4-26e8-4fd6-98d3-59adbef44c0d\"}]},\"type\":\"ConnectorPlacement.EquallySpacedConnector\",\"uuid\":\"5588d8d0-d459-45fe-a303-1ca6654e99d0\"}],\"packageUris\":[\"http://schema.mathworks.com/mf0/Connector/R2020b\"],\"version\":\"1.0\"}"
      mask Help: web([docroot '/physmod/simscape/ref/networkcouplerthermalmass.html'])
  Port 2 Interface1 : Subsystem  mask(Network Coupler (Thermal Mass) Port 2 Interface){}
      mask help: physmod:simscape:couplers:SimscapeNetworkCouplersLib:NetworkCouplerThermalMassPort2Interface_MD
      settings: PortSchema="{\"entries\":[{\"content\":{\"sides\":[{\"content\":{\"connectorIds\":[\"In1\",\"Out1\"]},\"type\":\"ConnectorPlacement.EquallySpacedRectSide\",\"uuid\":\"5a4c1550-e77d-42df-bf3e-b81963920de7\"},{\"content\":{\"connectorIds\":[\"RConn1\"],\"side\":\"RIGHT\"},\"type\":\"ConnectorPlacement.EquallySpacedRectSide\",\"uuid\":\"3fd730f7-5937-4563-a365-595aaae9027b\"},{\"content\":{\"connectorIds\":[],\"side\":\"TOP\"},\"type\":\"ConnectorPlacement.EquallySpacedRectSide\",\"uuid\":\"c16e04e4-26e8-4fd6-98d3-59adbef44c0d\"}]},\"type\":\"ConnectorPlacement.EquallySpacedConnector\",\"uuid\":\"5588d8d0-d459-45fe-a303-1ca6654e99d0\"}],\"packageUris\":[\"http://schema.mathworks.com/mf0/Connector/R2020b\"],\"version\":\"1.0\"}"
      mask Help: web([docroot '/physmod/simscape/ref/networkcouplerthermalmass.html'])
  Port 2 Interface2 : Subsystem  mask(Network Coupler (Thermal Mass) Port 2 Interface){}
      mask help: physmod:simscape:couplers:SimscapeNetworkCouplersLib:NetworkCouplerThermalMassPort2Interface_MD
      settings: PortSchema="{\"entries\":[{\"content\":{\"sides\":[{\"content\":{\"connectorIds\":[\"In1\",\"Out1\"]},\"type\":\"ConnectorPlacement.EquallySpacedRectSide\",\"uuid\":\"5a4c1550-e77d-42df-bf3e-b81963920de7\"},{\"content\":{\"connectorIds\":[\"RConn1\"],\"side\":\"RIGHT\"},\"type\":\"ConnectorPlacement.EquallySpacedRectSide\",\"uuid\":\"3fd730f7-5937-4563-a365-595aaae9027b\"},{\"content\":{\"connectorIds\":[],\"side\":\"TOP\"},\"type\":\"ConnectorPlacement.EquallySpacedRectSide\",\"uuid\":\"c16e04e4-26e8-4fd6-98d3-59adbef44c0d\"}]},\"type\":\"ConnectorPlacement.EquallySpacedConnector\",\"uuid\":\"5588d8d0-d459-45fe-a303-1ca6654e99d0\"}],\"packageUris\":[\"http://schema.mathworks.com/mf0/Connector/R2020b\"],\"version\":\"1.0\"}"
      mask Help: web([docroot '/physmod/simscape/ref/networkcouplerthermalmass.html'])
  Port 2 Interface3 : Subsystem  mask(Network Coupler (Voltage-Current) Port 2 Interface){}
      mask help: physmod:simscape:couplers:SimscapeNetworkCouplersLib:NetworkCouplerVoltageCurrentPort2Interface_MD
      settings: PortSchema="{\"entries\":[{\"content\":{\"sides\":[{\"content\":{\"connectorIds\":[\"In1\",\"Out1\"]},\"type\":\"ConnectorPlacement.EquallySpacedRectSide\",\"uuid\":\"5a4c1550-e77d-42df-bf3e-b81963920de7\"},{\"content\":{\"connectorIds\":[\"RConn1\"],\"side\":\"RIGHT\"},\"type\":\"ConnectorPlacement.EquallySpacedRectSide\",\"uuid\":\"3fd730f7-5937-4563-a365-595aaae9027b\"},{\"content\":{\"connectorIds\":[],\"side\":\"TOP\"},\"type\":\"ConnectorPlacement.EquallySpacedRectSide\",\"uuid\":\"c16e04e4-26e8-4fd6-98d3-59adbef44c0d\"}]},\"type\":\"ConnectorPlacement.EquallySpacedConnector\",\"uuid\":\"5588d8d0-d459-45fe-a303-1ca6654e99d0\"}],\"packageUris\":[\"http://schema.mathworks.com/mf0/Connector/R2020b\"],\"version\":\"1.0\"}"
      mask Help: web([docroot '/physmod/simscape/ref/networkcouplervoltagecurrent.html'])
  Rate Transition{,1..3} (4 alike) : RateTransition
  Rate transition (fast-to-slow){,1..3} (4 alike) : RateTransition  Integrity=off
  Rate transition (slow-to-fast){,1..3} (4 alike) : RateTransition  Integrity=off
  Solver Configuration1 : nesl_utility/Solver Configuration  PhysicalDomain=network_engine_domain  SubClassName=solver  LeftPortType=input  RightPortType=generic  Tones=[]  Harmonics=[]  SimulateNoise=off  Profile=off  UseLocalSampling=off  EnableSwitchedLinearOptims=on  FrequencyDomain=off  UseCCode=off  RelTol=0.001  AbsTol=1e-06  MinStep=1e-09  ToWorkspace=off  RevertToSquareIcSolve=off  NumHomotopyIterations=100  PhasorMode=off  PhasorModeNumHarmonics=1  DoDC=off  ResidualTolerance=1e-9  UseLocalSolver=on  LocalSolverChoice=NE_BACKWARD_EULER_ADVANCER  LocalSolverSampleTime=dt  DoFixedCost=on  MaxNonlinIter=3  MaxModeIter=2  ComputeImpulses=off  ImpulseIterations=2  LinearAlgebra=auto  EquationFormulation=NE_TIME_EF  DelaysMemoryBudget=1024  AutomaticFiltering=on  FilteringTimeConstant=0.001  PartitionStorageMethod=AS_NEEDED  PartitionMemoryBudget=1024  PartitionMethod=FAST
      settings: AttributesFormatString=Local Solver: %<UseLocalSolver>  SourceProductBaseCode=SS,PW,VE
  Solver Configuration2 : nesl_utility/Solver Configuration  PhysicalDomain=network_engine_domain  SubClassName=solver  LeftPortType=input  RightPortType=generic  Tones=[]  Harmonics=[]  SimulateNoise=off  Profile=off  UseLocalSampling=off  EnableSwitchedLinearOptims=on  FrequencyDomain=off  UseCCode=off  RelTol=0.001  AbsTol=1e-06  MinStep=1e-09  ToWorkspace=off  RevertToSquareIcSolve=off  NumHomotopyIterations=100  PhasorMode=off  PhasorModeNumHarmonics=1  DoDC=off  ResidualTolerance=1e-9  UseLocalSolver=on  LocalSolverChoice=NE_BACKWARD_EULER_ADVANCER  LocalSolverSampleTime=dt*5  DoFixedCost=on  MaxNonlinIter=3  MaxModeIter=2  ComputeImpulses=off  ImpulseIterations=2  LinearAlgebra=auto  EquationFormulation=NE_TIME_EF  DelaysMemoryBudget=1024  AutomaticFiltering=on  FilteringTimeConstant=0.001  PartitionStorageMethod=AS_NEEDED  PartitionMemoryBudget=1024  PartitionMethod=FAST
      settings: AttributesFormatString=Local Solver: %<UseLocalSolver>  SourceProductBaseCode=SS,PW,VE
  Solver Configuration3 : nesl_utility/Solver Configuration  PhysicalDomain=network_engine_domain  SubClassName=solver  LeftPortType=input  RightPortType=generic  Tones=[]  Harmonics=[]  SimulateNoise=off  Profile=off  UseLocalSampling=off  EnableSwitchedLinearOptims=on  FrequencyDomain=off  UseCCode=off  RelTol=0.001  AbsTol=1e-06  MinStep=1e-09  ToWorkspace=off  RevertToSquareIcSolve=off  NumHomotopyIterations=100  PhasorMode=off  PhasorModeNumHarmonics=1  DoDC=off  ResidualTolerance=1e-9  UseLocalSolver=on  LocalSolverChoice=NE_BACKWARD_EULER_ADVANCER  LocalSolverSampleTime=dt*2  DoFixedCost=on  MaxNonlinIter=3  MaxModeIter=2  ComputeImpulses=off  ImpulseIterations=2  LinearAlgebra=auto  EquationFormulation=NE_TIME_EF  DelaysMemoryBudget=1024  AutomaticFiltering=on  FilteringTimeConstant=0.001  PartitionStorageMethod=AS_NEEDED  PartitionMemoryBudget=1024  PartitionMethod=FAST
      settings: AttributesFormatString=Local Solver: %<UseLocalSolver>  SourceProductBaseCode=SS,PW,VE
  Unit Delay1 : UnitDelay  SampleTime=dt  HasFrameUpgradeWarning=on
  Vehicle Dynamics : Subsystem
  Vehicle Control : Subsystem  Tag=PublishSubsystem
      settings: PortSchema="{\"entries\":[{\"content\":{\"sides\":[{\"content\":{\"connectorIds\":[\"In1\"]},\"type\":\"ConnectorPlacement.EquallySpacedRectSide\",\"uuid\":\"b68a5c30-2a17-4a0c-a85e-064518f12190\"},{\"content\":{\"connectorIds\":[\"In2\",\"Out1\"],\"side\":\"RIGHT\"},\"type\":\"ConnectorPlacement.EquallySpacedRectSide\",\"uuid\":\"e14e894a-37e1-47c1-8ef8-e46ccf22e5bb\"},{\"content\":{\"connectorIds\":[],\"side\":\"TOP\"},\"type\":\"ConnectorPlacement.EquallySpacedRectSide\",\"uuid\":\"6e722464-54b7-4a5f-a776-dae3a11285e7\"}]},\"type\":\"ConnectorPlacement.EquallySpacedConnector\",\"uuid\":\"82601a10-23cc-4178-a2d7-02b0e1b6e975\"}],\"packageUris\":[\"http://schema.mathworks.com/mf0/Connector/R2020b\"],\"version\":\"1.0\"}"
  ZOH/1 : ZeroOrderHold  SampleTime=dt
  wires:
  Driver and Environment/3(Env) -> Rate Transition/1
  Port 2 Interface1/1(heat flow) -> Rate transition (slow-to-fast)1/1
  Rate Transition/1 -> Environment/1(T)
  Port 1 Interface2/1(temperature) -> Rate transition (fast-to-slow)2/1
  Port 2 Interface/1(heat flow) -> Rate transition (slow-to-fast)/1
  Rate transition (fast-to-slow)1/1 -> Port 2 Interface1/1(temperature)
  Port 1 Interface3/1(current) -> Rate transition (fast-to-slow)3/1
  Motor Drive/1(w) -> Rate Transition3/1
  Rate Transition2/1 -> Vehicle Dynamics/1(Test data)
  Rate transition (slow-to-fast)3/1 -> Port 1 Interface3/1(voltage)
  Rate transition (fast-to-slow)2/1 -> Port 2 Interface2/1(temperature)
  Rate transition (slow-to-fast)/1 -> Port 1 Interface/1(heat flow)
  Rate transition (slow-to-fast)2/1 -> Port 1 Interface2/1(heat flow)
  Driver and Environment/1(Veh) -> Rate Transition2/1
  Driver and Environment/2(ECU) -> Vehicle Control/1(ECU)
  Rate transition (fast-to-slow)/1 -> Port 2 Interface/1(temperature)
  Rate transition (fast-to-slow)3/1 -> Port 2 Interface3/1(current)
  Vehicle Control/1(iRef) -> Unit Delay1/1
  Port 1 Interface1/1(temperature) -> Rate transition (fast-to-slow)1/1
  Port 2 Interface2/1(heat flow) -> Rate transition (slow-to-fast)2/1
  ZOH/1/1 -> Vehicle Control/2(wMeas)
  Port 2 Interface3/1(voltage) -> Rate transition (slow-to-fast)3/1
  Port 1 Interface/1(temperature) -> Rate transition (fast-to-slow)/1
  Rate transition (slow-to-fast)1/1 -> Port 1 Interface1/1(heat flow)
  Rate Transition1/1 -> Motor Drive/1(iRef)
  Rate Transition3/1 -> ZOH/1/1
  Unit Delay1/1 -> Rate Transition1/1
  connections:
  Battery/LConn1 -- Port 1 Interface/LConn1
  Motor 1 Thermal Model/RConn1 -- Port 2 Interface2/RConn1
  Battery/RConn1 -- Port 2 Interface3/RConn1
  Motor Drive/LConn4 -- Port 1 Interface1/LConn1
  Cooling System/RConn1 -- Motor 1 Thermal Model/LConn1 -- Solver Configuration2/RConn1 -- Motor 2 Thermal Model/LConn1 -- Environment/RConn1
  Vehicle Dynamics/LConn1 -- Motor Drive/RConn1 -- Solver Configuration1/RConn1
  Cooling System/LConn1 -- Port 2 Interface/RConn1
  Motor Drive/LConn1 -- Port 1 Interface3/LConn1
  ERef2/LConn1 -- Motor Drive/LConn2
  Motor Drive/LConn3 -- Port 1 Interface2/LConn1
  Motor 2 Thermal Model/RConn1 -- Port 2 Interface1/RConn1
  Battery/LConn2 -- Solver Configuration3/RConn1 -- ERef1/LConn1
